simulink model "Rooftop_panel"  (R2015a)
settings: Solver=ode45  StartTime=0.0  StopTime=0.1  MaxStep=1e-6  RelTol=1e-3
InitFcn:
  | global Vpv_anterior;
  | global Ipv_anterior;
  | global Ppv_anterior;
  | global Vref;
  | 
  |  Vpv_anterior=60;
  | Ipv_anterior=0;
  | Ppv_anterior=0;
  | Vref=60;
libraries: powerlib x22, simulink x3, re_lib x1
settings Model: Creator=Juan  LastModifiedBy=Juan

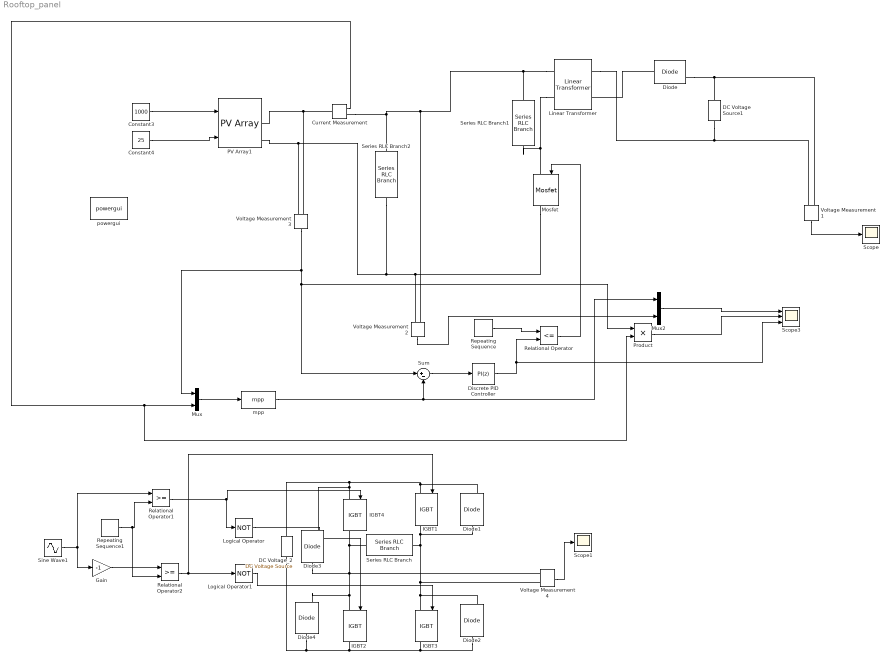
== system Rooftop_panel ==
  Constant3 : Constant  Value=1000
  Constant4 : Constant  Value=25
  Current Measurement : powerlib/Measurements/Current Measurement  PhasorSimulation=off  OutputType=Complex  PSBequivalent=0
  DC Voltage Source1 : powerlib/Electrical Sources/DC Voltage Source  Amplitude=450  Measurements=None
  DC Voltage_2 : powerlib/Electrical Sources/DC Voltage Source  Amplitude=450  Measurements=None
  Diode{,1..4} (5 alike) : powerlib/Power Electronics/Diode  Ron=0.001  Lon=0  Vf=0.8  IC=0  UseSnubber=off  Rs=500  Cs=250e-9  Measurements=on
  Discrete PID Controller : simulink/Continuous/PID Controller  Controller=PI  TimeDomain=Discrete-time  SampleTime=1e-4  IntegratorMethod=Forward Euler  FilterMethod=Forward Euler  Form=Parallel  UseFilter=on  ControllerParametersSource=internal  P=2e-4  I=2  D=0  N=100  InitialConditionSource=internal  InitialConditionForIntegrator=0  InitialConditionForFilter=0  ExternalReset=none  LimitOutput=off  UpperSaturationLimit=inf  LowerSaturationLimit=-inf  LinearizeAsGain=off  AntiWindupMode=none  Kb=1  TrackingMode=off  Kt=1  PParamMin=[]  PParamMax=[]  IParamMin=[]  IParamMax=[]  DParamMin=[]  DParamMax=[]  NParamMin=[]  NParamMax=[]  KbParamMin=[]  KbParamMax=[]  KtParamMin=[]  KtParamMax=[]  POutMin=[]  POutMax=[]  IOutMin=[]  IOutMax=[]  DOutMin=[]  DOutMax=[]  NOutMin=[]  NOutMax=[]  KbOutMin=[]  KbOutMax=[]  KtOutMin=[]  KtOutMax=[]  IntegratorOutMin=[]  IntegratorOutMax=[]  FilterOutMin=[]  FilterOutMax=[]  SumOutMin=[]  SumOutMax=[]  SumI1OutMin=[]  SumI1OutMax=[]  SumI2OutMin=[]  SumI2OutMax=[]  SumI3OutMin=[]  SumI3OutMax=[]  SumDOutMin=[]  SumDOutMax=[]  SaturationOutMin=[]  SaturationOutMax=[]  IntegratorContinuousStateAttributes=''  IntegratorStateMustResolveToSignalObject=off  IntegratorRTWStateStorageClass=Auto  FilterContinuousStateAttributes=''  FilterStateMustResolveToSignalObject=off  FilterRTWStateStorageClass=Auto  DifferentiatorICPrevScaledInput=0  DifferentiatorOutMin=[]  DifferentiatorOutMax=[]
  Gain : Gain  Gain=-1
  IGBT{1..4} (4 alike) : powerlib/Power Electronics/IGBT  Ron=0.001  Lon=0  Vf=1  Tf=1e-6  Tt=2e-6  IC=0  Rs=1e5  Cs=inf  Measurements=on
  Linear Transformer : powerlib/Elements/Linear Transformer  UNITS=SI  NominalPower=[ 10e3 10e3 ]  winding1=[60 0.002 0]  winding2=[450 0.002 0]  ThreeWindings=off  winding3=[3.15e+05 0.7938 0.084225]  RmLm=[1.0e+06 0]  Measurements=None  DataType=on
  Logical Operator : Logic  Operator=NOT  AllPortsSameDT=off  OutDataTypeStr=boolean
  Logical Operator1 : Logic  Operator=NOT  AllPortsSameDT=off  OutDataTypeStr=boolean
  Mosfet : powerlib/Power Electronics/Mosfet  Ron=0.1  Lon=0  Rd=0.01  Vfd=0  IC=0  Rs=1e5  Cs=inf  Measurements=on
  Mux : Mux  Inputs=2
  Mux2 : Mux  Inputs=2
  PV Array1 : re_lib/Solar/PV Array  Npar=1  Nser=2  PlotType=array @ 1000 W/m2 & specified temperatures  S_vec="[ 1000  500  100 ]"  Temp_C_vec="[ 45 25  ]"  ModuleName=1Soltech 1STH-215-P  PlotWhenSelected=off  Pm=213.15  Ncell=60  Voc=36.3  Isc=7.84  Vm=29  Im=7.35  beta_Voc_pc=-0.36099  alpha_Isc_pc=0.102  beta_Voc=-0.13104  alpha_Isc=0.007997  IL=7.8649  I0=2.9259e-10  nI=0.98117  Rsh=313.3991  Rs=0.39383  BAL=off  Tc=1e-6  Tfilter=5e-5
  Product : Product
  Relational Operator : RelationalOperator  Operator=<=  OutDataTypeStr=boolean
  Relational Operator1 : RelationalOperator  OutDataTypeStr=boolean
  Relational Operator2 : RelationalOperator  OutDataTypeStr=boolean
  Repeating Sequence : simulink/Sources/Repeating Sequence  rep_seq_t=[0 1e-4]  rep_seq_y=[0 1]
  Repeating Sequence1 : simulink/Sources/Repeating Sequence  rep_seq_t=[0 50e-6 100e-6]  rep_seq_y=[-1 1 -1]
  Scope : Scope
      settings: YMin=0.05  YMax=0.525
  Scope1 : Scope
      settings: YMin=-40000  YMax=40000
  Scope3 : Scope  NumInputPorts=3
      settings: YMin=42.5~-5~-5  YMax=72.5~5~5  SaveName=ScopeData3
  Series RLC Branch : powerlib/Elements/Series RLC Branch  LConnTagsString=__new0  RConnTagsString=__new0  BranchType=RL  Resistance=30  Inductance=5e-3  SetiL0=off  InitialCurrent=0  Capacitance=1e-6  Setx0=off  InitialVoltage=0  Measurements=None
  Series RLC Branch1 : powerlib/Elements/Series RLC Branch  LConnTagsString=__new0  RConnTagsString=__new0  BranchType=L  Resistance=0  Inductance=5e-3  SetiL0=off  InitialCurrent=0  Capacitance=inf  Setx0=off  InitialVoltage=0  Measurements=None
  Series RLC Branch2 : powerlib/Elements/Series RLC Branch  LConnTagsString=__new0  RConnTagsString=__new0  BranchType=C  Resistance=0  Inductance=5e-3  SetiL0=off  InitialCurrent=0  Capacitance=500e-6  Setx0=off  InitialVoltage=0  Measurements=None
  Sine Wave1 : Sin  Amplitude=250/450  Frequency=2*pi*50  SampleTime=0
  Sum : Sum  Inputs=|+-
  Voltage Measurement{1..4} (4 alike) : powerlib/Measurements/Voltage Measurement  PhasorSimulation=off  OutputType=Complex  PSBequivalent=0
  mpp : S-Function  FunctionName=mpp
  powergui : powerlib/powergui  Priority=1  SimulationMode=Discrete  SolverType=Tustin/Backward Euler (TBE)  SampleTime=1e-6  frequency=60  SPID=off  DisableSnubberDevices=off  DisableRonSwitches=off  DisableVfSwitches=off  SwTol=0  DisplayEquations=off  Interpol=off  methode=off  Ts=100  FunctionMessages=off  echomessages=off  HookPort=off  EnableUseOfTLC=off  x0status=blocks  frequencyindice=0  Pbase=100e6  ErrMax=1e-4  Iterations=50  UnitsV=kV  UnitsW=MW  buscounter=0  RestoreLinks=warning  ResistiveCurrentMeasurement=off  Frange=[0:2:500]  Ylog=off  Xlog=on  ShowGrid=off  save=off  variable=ZData  structure=0  ZoomFFT=off  StartTime=0.0  cycles=1  DisplayStyle=1  fundamental=60  FreqAxis=off  MaxFrequency=1000  frequencyindicesteady=1  RmsSteady=1  display=off
  wires:
  Repeating Sequence/1 -> Relational Operator/1
  Relational Operator/1 -> Mosfet/1
  Voltage Measurement2/1 -> Mux2/2
  Discrete PID Controller/1 -> Scope3/3, Relational Operator/2
  Sum/1 -> Discrete PID Controller/1
  Voltage Measurement1/1 -> Scope/1
  Constant4/1 -> PV Array1/2
  Constant3/1 -> PV Array1/1
  mpp/1 -> Mux2/1, Sum/2
  Mux/1 -> mpp/1
  Voltage Measurement3/1 -> Mux/1, Product/1, Sum/1
  Current Measurement/1 -> Product/2, Mux/2
  Mux2/1 -> Scope3/1
  Product/1 -> Scope3/2
  Voltage Measurement4/1 -> Scope1/1
  Repeating Sequence1/1 -> Relational Operator2/2, Relational Operator1/2
  Relational Operator1/1 -> IGBT4/1, Logical Operator/1
  Relational Operator2/1 -> IGBT1/1, Logical Operator1/1
  Sine Wave1/1 -> Gain/1, Relational Operator1/1
  Logical Operator/1 -> IGBT2/1
  Logical Operator1/1 -> IGBT3/1
  Gain/1 -> Relational Operator2/1
  connections:
  Diode/RConn1 -- Voltage Measurement1/LConn1 -- DC Voltage Source1/RConn1
  Linear Transformer/RConn1 -- Voltage Measurement1/LConn2 -- DC Voltage Source1/LConn1
  Diode/LConn1 -- Linear Transformer/RConn2
  Linear Transformer/LConn1 -- Current Measurement/RConn1 -- Series RLC Branch2/LConn1 -- Voltage Measurement2/LConn1 -- Series RLC Branch1/RConn1
  Linear Transformer/LConn2 -- Mosfet/LConn1 -- Series RLC Branch1/LConn1
  Mosfet/RConn1 -- Voltage Measurement3/LConn2 -- PV Array1/RConn2 -- Series RLC Branch2/RConn1 -- Voltage Measurement2/LConn2
  PV Array1/RConn1 -- Current Measurement/LConn1 -- Voltage Measurement3/LConn1
  IGBT4/RConn1 -- Series RLC Branch/LConn1 -- Voltage Measurement4/LConn1 -- Diode3/LConn1 -- Diode4/RConn1 -- IGBT2/LConn1
  IGBT1/RConn1 -- Diode1/LConn1 -- Voltage Measurement4/LConn2 -- Diode2/RConn1 -- IGBT3/LConn1 -- Series RLC Branch/RConn1
  IGBT1/LConn1 -- Diode1/RConn1 -- Diode3/RConn1 -- IGBT4/LConn1 -- DC Voltage_2/RConn1
  IGBT2/RConn1 -- Diode4/LConn1 -- DC Voltage_2/LConn1 -- Diode2/LConn1 -- IGBT3/RConn1
